simulink model "SVPWMtrialsweird"  (R2015b)
settings: Solver=VariableStepAuto  StartTime=0.0  StopTime=0.05  RelTol=1e-3
libraries: powerlib x29, simulink x1
(part 1 of 2)
settings Model: Creator=hakan  LastModifiedBy=hakan

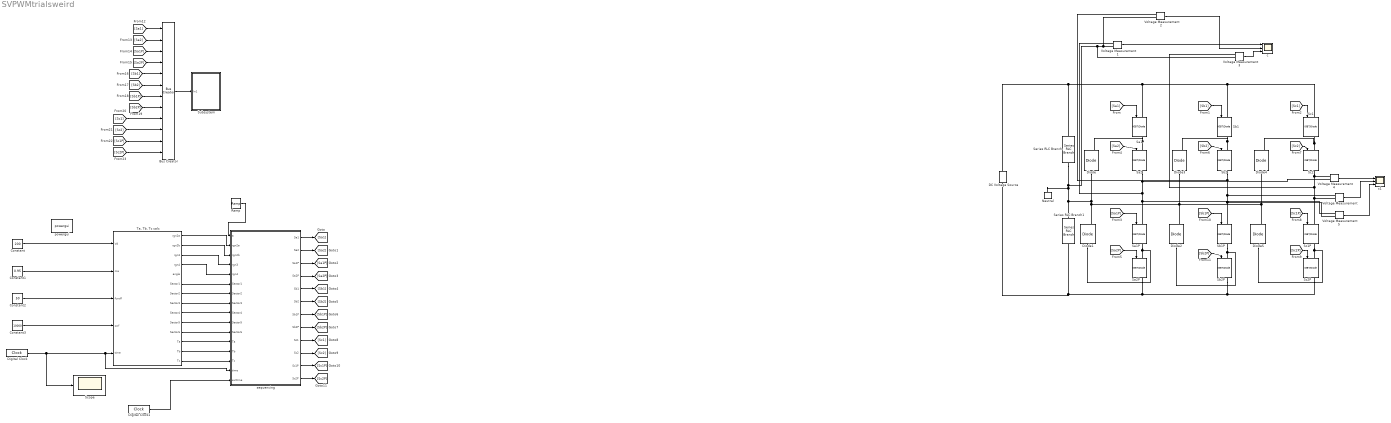
== system SVPWMtrialsweird ==
  Bus Creator : BusCreator  Inputs=12
  Constant : Constant  Value=200
  Constant1 : Constant  Value=0.95
  Constant2 : Constant  Value=50
  Constant3 : Constant  Value=10000  VectorParams1D=off
  DC Voltage Source : powerlib/Electrical Sources/DC Voltage Source  Amplitude=100  Measurements=None
  Digital Clock : DigitalClock  SampleTime=0.00001
  Digital Clock1 : DigitalClock  SampleTime=0.000001
  Diode{,1..5} (6 alike) : powerlib/Power Electronics/Diode  Ron=0.001  Lon=0  Vf=0.8  IC=0  UseSnubber=off  Rs=500  Cs=250e-9  Measurements=on
  Neutral : powerlib/Elements/Neutral  LConnTagsString=a  NodeNumber=10
  Ramp : simulink/Sources/Ramp  slope=1  start=0  X0=0
  "Sa1 " : powerlib/Power Electronics/IGBT//Diode  Ron=1e-3  Rs=1e5  Cs=inf  Measurements=on
  Sa1P : powerlib/Power Electronics/IGBT//Diode  Ron=1e-3  Rs=1e5  Cs=inf  Measurements=on
  Sa2 : powerlib/Power Electronics/IGBT//Diode  Ron=1e-3  Rs=1e5  Cs=inf  Measurements=on
  Sa2P : powerlib/Power Electronics/IGBT//Diode  Ron=1e-3  Rs=1e5  Cs=inf  Measurements=on
  Sb1 : powerlib/Power Electronics/IGBT//Diode  Ron=1e-3  Rs=1e5  Cs=inf  Measurements=on
  Sb1P : powerlib/Power Electronics/IGBT//Diode  Ron=1e-3  Rs=1e5  Cs=inf  Measurements=on
  Sb2 : powerlib/Power Electronics/IGBT//Diode  Ron=1e-3  Rs=1e5  Cs=inf  Measurements=on
  Sb2P : powerlib/Power Electronics/IGBT//Diode  Ron=1e-3  Rs=1e5  Cs=inf  Measurements=on
  Sc1 : powerlib/Power Electronics/IGBT//Diode  Ron=1e-3  Rs=1e5  Cs=inf  Measurements=on
  Sc1P : powerlib/Power Electronics/IGBT//Diode  Ron=1e-3  Rs=1e5  Cs=inf  Measurements=on
  Sc2 : powerlib/Power Electronics/IGBT//Diode  Ron=1e-3  Rs=1e5  Cs=inf  Measurements=on
  Sc2P : powerlib/Power Electronics/IGBT//Diode  Ron=1e-3  Rs=1e5  Cs=inf  Measurements=on
  Scope : Scope
  Series RLC Branch : powerlib/Elements/Series RLC Branch  LConnTagsString=__new0  RConnTagsString=__new0  BranchType=RC  Resistance=1  Inductance=1e-3  SetiL0=off  InitialCurrent=0  Capacitance=1000e-6  Setx0=off  InitialVoltage=0  Measurements=None
  Series RLC Branch1 : powerlib/Elements/Series RLC Branch  LConnTagsString=__new0  RConnTagsString=__new0  BranchType=RC  Resistance=1  Inductance=1e-3  SetiL0=off  InitialCurrent=0  Capacitance=1000e-6  Setx0=off  InitialVoltage=0  Measurements=None
  Subsystem : Subsystem
  "Ta, Tb, Tc calc" : MATLAB Function  TreatAsAtomicUnit=on
  Voltage Measurement{,1..5} (6 alike) : powerlib/Measurements/Voltage Measurement  PhasorSimulation=off  OutputType=Complex  PSBequivalent=0
  c : Scope  NumInputPorts=3
  c1 : Scope  NumInputPorts=3
  powergui : powerlib/powergui  Priority=1  SimulationMode=Continuous  SolverType=Tustin/Backward Euler (TBE)  SampleTime=50e-6  frequency=60  SPID=off  DisableSnubberDevices=off  DisableRonSwitches=off  DisableVfSwitches=off  SwTol=0  DisplayEquations=off  Interpol=off  ExternalGateDelay=off  methode=off  Ts=10  FunctionMessages=off  echomessages=off  HookPort=off  EnableUseOfTLC=off  x0status=blocks  frequencyindice=0  Pbase=100e6  ErrMax=1e-4  Iterations=50  UnitsV=kV  UnitsW=MW  buscounter=0  RestoreLinks=warning  ResistiveCurrentMeasurement=off  Frange=[0:2:500]  Ylog=off  Xlog=on  ShowGrid=off  save=off  variable=ZData  structure=dutycycles  ZoomFFT=off  StartTime=0.0  cycles=1  DisplayStyle=1  fundamental=5000  FreqAxis=off  MaxFrequency=10000  frequencyindicesteady=1  RmsSteady=1  display=off
  sequencing : MATLAB Function  TreatAsAtomicUnit=on
  wires:
  Constant/1 -> "Ta, Tb, Tc calc"/1(Vd)
  Constant1/1 -> "Ta, Tb, Tc calc"/2(ma)
  Constant2/1 -> "Ta, Tb, Tc calc"/3(fundf)
  Constant3/1 -> "Ta, Tb, Tc calc"/4(swf)
  "Ta, Tb, Tc calc"/6(Sector1) -> sequencing/6(Sector1)
  "Ta, Tb, Tc calc"/7(Sector2) -> sequencing/7(Sector2)
  "Ta, Tb, Tc calc"/8(Sector3) -> sequencing/8(Sector3)
  "Ta, Tb, Tc calc"/9(Sector4) -> sequencing/9(Sector4)
  "Ta, Tb, Tc calc"/11(Sector6) -> sequencing/11(Sector6)
  "Ta, Tb, Tc calc"/10(Sector5) -> sequencing/10(Sector5)
  "Ta, Tb, Tc calc"/12(Ta) -> sequencing/12(Ta)
  "Ta, Tb, Tc calc"/13(Tb) -> sequencing/13(Tb)
  "Ta, Tb, Tc calc"/14(Tc) -> sequencing/14(Tc)
  Digital Clock/1 -> sequencing/15(time), "Ta, Tb, Tc calc"/5(time), Scope/1
  Bus Creator/1 -> Subsystem/1(In1)
  sequencing/1(Sa1) -> [Sa1]
  sequencing/2(Sa2) -> [Sa2]
  sequencing/3(Sa1P) -> [Sa1P]
  sequencing/4(Sa2P) -> [Sa2P]
  sequencing/5(Sb1) -> [Sb1]
  sequencing/6(Sb2) -> [Sb2]
  sequencing/7(Sb1P) -> [Sb1P]
  sequencing/8(Sb2P) -> [Sb2P]
  sequencing/9(Sc1) -> [Sc1]
  sequencing/10(Sc2) -> [Sc2]
  sequencing/11(Sc1P) -> [Sc1P]
  sequencing/12(Sc2P) -> [Sc2P]
  [Sa1] -> "Sa1 "/1
  [Sa1P] -> Sa1P/1
  [Sa2] -> Sa2/1
  [Sa2P] -> Sa2P/1
  [Sb1] -> Sb1/1
  [Sb2] -> Sb2/1
  [Sb1P] -> Sb1P/1
  [Sb2P] -> Sb2P/1
  [Sc2P] -> Sc2P/1
  [Sc1P] -> Sc1P/1
  [Sc1] -> Sc1/1
  [Sc2] -> Sc2/1
  [Sa1] -> Bus Creator/1
  [Sa2] -> Bus Creator/2
  [Sa1P] -> Bus Creator/3
  [Sa2P] -> Bus Creator/4
  [Sb1] -> Bus Creator/5
  [Sb2] -> Bus Creator/6
  [Sb1P] -> Bus Creator/7
  [Sb2P] -> Bus Creator/8
  [Sc1] -> Bus Creator/9
  [Sc2] -> Bus Creator/10
  [Sc1P] -> Bus Creator/11
  [Sc2P] -> Bus Creator/12
  Digital Clock1/1 -> sequencing/16(exttime)
  Ramp/1 -> sequencing/1(a)
  "Ta, Tb, Tc calc"/4(rgn4) -> sequencing/5(rgn4)
  "Ta, Tb, Tc calc"/3(rgn3) -> sequencing/4(rgn3)
  "Ta, Tb, Tc calc"/2(rgn2b) -> sequencing/3(rgn2b)
  "Ta, Tb, Tc calc"/1(rgn2a) -> sequencing/2(rgn2a)
  Voltage Measurement3/1 -> c/3
  Voltage Measurement1/1 -> c/1
  Voltage Measurement2/1 -> c/2
  Voltage Measurement4/1 -> c1/1
  Voltage Measurement/1 -> c1/2
  Voltage Measurement5/1 -> c1/3
  connections:
  DC Voltage Source/RConn1 -- Sc1/LConn1 -- Sb1/LConn1 -- "Sa1 "/LConn1 -- Series RLC Branch/LConn1
  DC Voltage Source/LConn1 -- Sb2P/RConn1 -- Sc2P/RConn1 -- Sa2P/RConn1 -- Series RLC Branch1/RConn1
  "Sa1 "/RConn1 -- Diode/RConn1 -- Sa2/LConn1
  Sa2/RConn1 -- Voltage Measurement4/LConn2 -- Voltage Measurement1/LConn1 -- Voltage Measurement5/LConn1 -- Sa1P/LConn1
  Sa1P/RConn1 -- Diode1/LConn1 -- Sa2P/LConn1
  Sb1/RConn1 -- Diode3/RConn1 -- Sb2/LConn1
  Sb2/RConn1 -- Voltage Measurement2/LConn1 -- Voltage Measurement/LConn1 -- Sb1P/LConn1 -- Voltage Measurement5/LConn2
  Sb1P/RConn1 -- Diode2/LConn1 -- Sb2P/LConn1
  Sc1/RConn1 -- Diode4/RConn1 -- Sc2/LConn1
  Sc2/RConn1 -- Voltage Measurement4/LConn1 -- Voltage Measurement3/LConn1 -- Sc1P/LConn1 -- Voltage Measurement/LConn2
  Sc1P/RConn1 -- Diode5/LConn1 -- Sc2P/LConn1
  Diode/LConn1 -- Diode3/LConn1 -- Diode5/RConn1 -- Diode4/LConn1 -- Diode2/RConn1 -- Diode1/RConn1 -- Voltage Measurement2/LConn2 -- Voltage Measurement1/LConn2 -- Voltage Measurement3/LConn2 -- Series RLC Branch/RConn1 -- Neutral/LConn1 -- Series RLC Branch1/LConn1

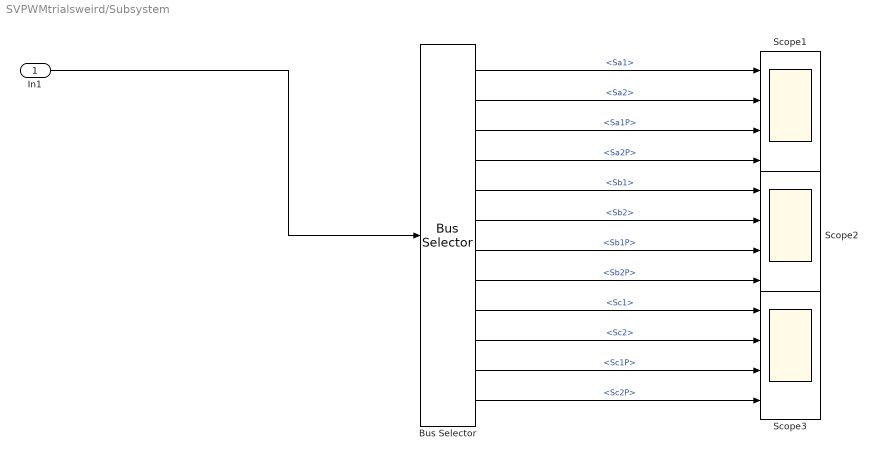
== system SVPWMtrialsweird/Subsystem ==
  In1 : Inport
  Bus Selector : BusSelector  OutputSignals=Sa1,Sa2,Sa1P,Sa2P,Sb1,Sb2,Sb1P,Sb2P,Sc1,Sc2,Sc1P,Sc2P
  Scope1 : Scope  NumInputPorts=4
  Scope2 : Scope  NumInputPorts=4
  Scope3 : Scope  NumInputPorts=4
  wires:
  In1/1 -> Bus Selector/1
  Bus Selector/4 -> Scope1/4  "<Sa2P>"
  Bus Selector/3 -> Scope1/3  "<Sa1P>"
  Bus Selector/2 -> Scope1/2  "<Sa2>"
  Bus Selector/1 -> Scope1/1  "<Sa1>"
  Bus Selector/5 -> Scope2/1  "<Sb1>"
  Bus Selector/6 -> Scope2/2  "<Sb2>"
  Bus Selector/7 -> Scope2/3  "<Sb1P>"
  Bus Selector/8 -> Scope2/4  "<Sb2P>"
  Bus Selector/9 -> Scope3/1  "<Sc1>"
  Bus Selector/12 -> Scope3/4  "<Sc2P>"
  Bus Selector/11 -> Scope3/3  "<Sc1P>"
  Bus Selector/10 -> Scope3/2  "<Sc2>"

== matlab function SVPWMtrialsweird/Ta, Tb, Tc calc ==
  data: rgn2a output; rgn2b output; rgn3 output; rgn4 output; Vd input; ma input; fundf input; angle output; swf input; time input; Sector1 output; Sector2 output; Sector3 output; Sector4 output; Sector5 output; Sector6 output; Ta output; Tb output; Tc output
function [rgn2a, rgn2b, rgn3, rgn4, angle, Sector1, Sector2, Sector3, Sector4, Sector5,Sector6, Ta, Tb, Tc] = fcn(Vd,ma,fundf, swf, time)
% this program works for magnitude of Vref is greater then Vd/3 meaning ma
% must be greater than 1/sqrt(3). for smaller ma's computation is a bit
% more tricky therefore it is omitted for simplicity for now. 
%#ok<*NASGU>
Vref = ma*Vd/sqrt(3); %magnitude of Vref
theta = 2*pi*fundf*time; %angle of Vref
angle = mod(theta, 2*pi);
Ts = 1/swf;
Ta = 0;
Tb = 0;
Tc = 0;
output = 0;
Sector1 = 0; Sector2 = 0; Sector3 = 0; Sector4= 0; Sector5 = 0; Sector6 = 0;
rgn2a = 0 ;rgn2b = 0; rgn3 = 0; rgn4 = 0;
% Sa1=0; Sa2=0; Sa1P=0; Sa2P=0; Sb1=0; Sb2=0; Sb1P=0; Sb2P=0; Sc1=0; Sc2=0; Sc1P=0; Sc2P=0;
anglefrom3to2= 0 ;
%% Sector 1


if (mod(theta, 2*pi)<=pi/3)&&(mod(theta, 2*pi)>0)  % sector 1

    n = 1;
    thetaprime = angle - (n-1)*pi/3;
        for aci = 0:0.00001:pi/3   
            la = sqrt(3)*cos(aci)-sin(aci);
                if (la*ma > 0.99)&&(la*ma<=1)
                    anglefrom3to2 = aci; %leaving angle from region 3 to region 2
                    break
                end
        end

    %anglefrom3to2 = asin(1-1/(sqrt(3)*ma)); 
    anglefrom2to4 = pi/3 - anglefrom3to2; %leaving angle from region 2 to region 4
    if (mod(theta, 2*pi)<=anglefrom3to2) % then sector 1 region 3
        rgn2a = 0 ;rgn2b = 0; rgn3 = 1; rgn4 = 0;
        Ta = Ts*(2-2*ma*sin(pi/3+thetaprime));
        Tb = Ts*2*ma*sin(thetaprime);
        Tc = Ts*(2*ma*sin(pi/3-thetaprime)-1);        
    else if (mod(theta,2*pi)>anglefrom3to2)&&(mod(theta,2*pi)<=anglefrom2to4) % then sector 1 region 2
            if angle<= pi/6 % then 2a
                rgn2a= 1; rgn2b = 0; rgn3 = 0; rgn4=0;
            else % then 2b
                rgn2a= 0; rgn2b = 1; rgn3 = 0; rgn4=0;
            end
            Ta = Ts*(1-2*ma*sin(thetaprime));
            Tb = Ts*(2*ma*sin(pi/3+thetaprime)-1);
            Tc = Ts*(1-2*ma*sin(pi/3-thetaprime));       
        else if (mod(theta,2*pi)>anglefrom2to4) % then sector 1 region 4
               rgn2a = 0 ;rgn2b = 0; rgn3 = 0; rgn4 = 1;
               Ta = Ts*(2*ma*sin(thetaprime)-1);
               Tb = Ts*(2*ma*sin(pi/3-thetaprime));
               Tc = Ts*(2-2*ma*sin(pi/3+thetaprime));               
            end
        end
    end
    Sector1 = 1; Sector2 = 0; Sector3 = 0; Sector4= 0; Sector5 = 0; Sector6 = 0;
end
%% Sector 2


if (mod(theta, 2*pi)<=2*pi/3)&&(mod(theta, 2*pi)>pi/3)  % sector 2
    
    n = 2;
    thetaprime = angle - (n-1)*pi/3;
        for aci = 0:0.00001:pi/3   
            la = sqrt(3)*cos(aci)-sin(aci);
                if (la*ma > 0.99)&&(la*ma<=1)
                    anglefrom3to2 = aci+pi/3; %leaving angle from region 3 to region 2
                    break
                end
        end
    %anglefrom3to2 = pi/3 + asin(1-1/(sqrt(3)*ma));
    anglefrom2to4 = pi/3 + pi/3 - anglefrom3to2;
    if (mod(theta, 2*pi)<=anglefrom3to2) % then sector 2 region 3
        rgn2a = 0 ;rgn2b = 0; rgn3 = 1; rgn4 = 0;
        Ta = Ts*(2-2*ma*sin(pi/3+thetaprime));
        Tb = Ts*2*ma*sin(thetaprime);
        Tc = Ts*(2*ma*sin(pi/3-thetaprime)-1); 
    else if (mod(theta,2*pi)>anglefrom3to2)&&(mod(theta,2*pi)<=anglefrom2to4) % then sector 2 region 2
            if angle<=pi/2 %then 2a
                rgn2a= 1; rgn2b = 0; rgn3 = 0; rgn4=0;
            else % then 2b
                rgn2a= 0; rgn2b = 1; rgn3 = 0; rgn4=0;
            end
            Ta = Ts*(1-2*ma*sin(thetaprime));
            Tb = Ts*(2*ma*sin(pi/3+thetaprime)-1);
            Tc = Ts*(1-2*ma*sin(pi/3-thetaprime)); 
        else if (mod(theta,2*pi)>anglefrom2to4) % then sector 2 region 4
               rgn2a = 0 ;rgn2b = 0; rgn3 = 0; rgn4 = 1;
               Ta = Ts*(2*ma*sin(thetaprime)-1);
               Tb = Ts*(2*ma*sin(pi/3-thetaprime));
               Tc = Ts*(2-2*ma*sin(pi/3+thetaprime)); 
            end
        end
    end
    Sector1 = 0; Sector2 = 1; Sector3 = 0; Sector4= 0; Sector5 = 0; Sector6 = 0;
end
%% Sector 3

if (mod(theta, 2*pi)<=pi)&&(mod(theta, 2*pi)>2*pi/3)  % sector 3
    
    n = 3;
    thetaprime = angle - (n-1)*pi/3;
        for aci = 0:0.00001:pi/3   
            la = sqrt(3)*cos(aci)-sin(aci);
                if (la*ma > 0.99)&&(la*ma<=1)
                    anglefrom3to2 = aci+pi/3+pi/3; %leaving angle from region 3 to region 2
                    break
                end
        end    
    %anglefrom3to2 = 2*pi/3 + asin(1-1/(sqrt(3)*ma));
    anglefrom2to4 = 2*pi/3 + pi/3 - anglefrom3to2;
    if (mod(theta, 2*pi)<=anglefrom3to2) % then sector 3 region 3
        rgn2a = 0 ;rgn2b = 0; rgn3 = 1; rgn4 = 0;
        Ta = Ts*(2-2*ma*sin(pi/3+thetaprime));
        Tb = Ts*2*ma*sin(thetaprime);
        Tc = Ts*(2*ma*sin(pi/3-thetaprime)-1); 
    else if (mod(theta,2*pi)>anglefrom3to2)&&(mod(theta,2*pi)<=anglefrom2to4) % then sector 3 region 2
            if angle<=5*pi/6 %then 2a
                rgn2a= 1; rgn2b = 0; rgn3 = 0; rgn4=0;
            else % then 2b
                rgn2a= 0; rgn2b = 1; rgn3 = 0; rgn4=0;
            end
            Ta = Ts*(1-2*ma*sin(thetaprime));
            Tb = Ts*(2*ma*sin(pi/3+thetaprime)-1);
            Tc = Ts*(1-2*ma*sin(pi/3-thetaprime)); 
        else if (mod(theta,2*pi)>anglefrom2to4) % then sector 3 region 4
                rgn2a = 0 ;rgn2b = 0; rgn3 = 0; rgn4 = 1;
               Ta = Ts*(2*ma*sin(thetaprime)-1);
               Tb = Ts*(2*ma*sin(pi/3-thetaprime));
               Tc = Ts*(2-2*ma*sin(pi/3+thetaprime)); 
            end
        end
    end
    Sector1 = 0; Sector2 = 0; Sector3 = 1; Sector4= 0; Sector5 = 0; Sector6 = 0;
end

%% Sector 4


if (mod(theta, 2*pi)<=4*pi/3)&&(mod(theta, 2*pi)>pi)  % sector 4
    

    n = 4;
    thetaprime = angle - (n-1)*pi/3;
        for aci = 0:0.00001:pi/3   
            la = sqrt(3)*cos(aci)-sin(aci);
                if (la*ma > 0.99)&&(la*ma<=1)
                    anglefrom3to2 = aci+pi/3+pi/3+pi/3; %leaving angle from region 3 to region 2
                    break
                end
        end    
    %anglefrom3to2 = pi + asin(1-1/(sqrt(3)*ma));
    anglefrom2to4 = pi + pi/3 - anglefrom3to2;
    if (mod(theta, 2*pi)<=anglefrom3to2) % then sector 4 region 3
        rgn2a = 0 ;rgn2b = 0; rgn3 = 1; rgn4 = 0;
        Ta = Ts*(2-2*ma*sin(pi/3+thetaprime));
        Tb = Ts*2*ma*sin(thetaprime);
        Tc = Ts*(2*ma*sin(pi/3-thetaprime)-1); 
    else if (mod(theta,2*pi)>anglefrom3to2)&&(mod(theta,2*pi)<=anglefrom2to4) % then sector 4 region 2
            if angle<=7*pi/6 %then 2a
                rgn2a= 1; rgn2b = 0; rgn3 = 0; rgn4=0;
            else % then 2b
                rgn2a= 0; rgn2b = 1; rgn3 = 0; rgn4=0;
            end
            Ta = Ts*(1-2*ma*sin(thetaprime));
            Tb = Ts*(2*ma*sin(pi/3+thetaprime)-1);
            Tc = Ts*(1-2*ma*sin(pi/3-thetaprime));
        else if (mod(theta,2*pi)>anglefrom2to4) % then sector 4 region 4
                rgn2a = 0 ;rgn2b = 0; rgn3 = 0; rgn4 = 1;
               Ta = Ts*(2*ma*sin(thetaprime)-1);
               Tb = Ts*(2*ma*sin(pi/3-thetaprime));
               Tc = Ts*(2-2*ma*sin(pi/3+thetaprime)); 
            end
        end
    end
    Sector1 = 0; Sector2 = 0; Sector3 = 0; Sector4= 1; Sector5 = 0; Sector6 = 0;
end
%% Sector 5 

if (mod(theta, 2*pi)<=5*pi/3)&&(mod(theta, 2*pi)>4*pi/3)  % sector 5
    
    n = 5;
    thetaprime = angle - (n-1)*pi/3;
    %anglefrom3to2 = 4*pi/3 + asin(1-1/(sqrt(3)*ma));
        for aci = 0:0.00001:pi/3   
            la = sqrt(3)*cos(aci)-sin(aci);
                if (la*ma > 0.99)&&(la*ma<=1)
                    anglefrom3to2 = aci+pi/3+pi/3+pi/3+pi/3; %leaving angle from region 3 to region 2
                    break
                end
        end    
    anglefrom2to4 = 4*pi/3 + pi/3 - anglefrom3to2;
    if (mod(theta, 2*pi)<=anglefrom3to2) % then sector 5 region 3
        rgn2a = 0 ;rgn2b = 0; rgn3 = 1; rgn4 = 0;
        Ta = Ts*(2-2*ma*sin(pi/3+thetaprime));
        Tb = Ts*2*ma*sin(thetaprime);
        Tc = Ts*(2*ma*sin(pi/3-thetaprime)-1); 
    else if (mod(theta,2*pi)>anglefrom3to2)&&(mod(theta,2*pi)<=anglefrom2to4) % then sector 5 region 2
            if angle<=3*pi/2 %then 2a
                rgn2a= 1; rgn2b = 0; rgn3 = 0; rgn4=0;
            else % then 2b
                rgn2a= 0; rgn2b = 1; rgn3 = 0; rgn4=0;
            end
            Ta = Ts*(1-2*ma*sin(thetaprime));
            Tb = Ts*(2*ma*sin(pi/3+thetaprime)-1);
            Tc = Ts*(1-2*ma*sin(pi/3-thetaprime));
        else if (mod(theta,2*pi)>anglefrom2to4) % then sector 5 region 4
               rgn2a = 0 ;rgn2b = 0; rgn3 = 0; rgn4 = 1;
               Ta = Ts*(2*ma*sin(thetaprime)-1);
               Tb = Ts*(2*ma*sin(pi/3-thetaprime));
               Tc = Ts*(2-2*ma*sin(pi/3+thetaprime)); 
            end
        end
    end
    Sector1 = 0; Sector2 = 0; Sector3 = 0; Sector4= 0; Sector5 = 1; Sector6 = 0;
end

%% Sector 6 

if (mod(theta, 2*pi)<=2*pi)&&(mod(theta, 2*pi)>5*pi/3)  % sector 6
    
    n = 6;
    thetaprime = angle - (n-1)*pi/3;
        for aci = 0:0.00001:pi/3   
            la = sqrt(3)*cos(aci)-sin(aci);
                if (la*ma > 0.99)&&(la*ma<=1)
                    anglefrom3to2 = aci+pi/3+pi/3+pi/3+pi/3+pi/3; %leaving angle from region 3 to region 2
                    break
                end
        end    
    %anglefrom3to2 = 5*pi/3 + asin(1-1/(sqrt(3)*ma));
    anglefrom2to4 = 5*pi/3 + pi/3 - anglefrom3to2;
    if (mod(theta, 2*pi)<=anglefrom3to2) % then sector 6 region 3
        rgn2a = 0 ;rgn2b = 0; rgn3 = 1; rgn4 = 0;
        Ta = Ts*(2-2*ma*sin(pi/3+thetaprime));
        Tb = Ts*2*ma*sin(thetaprime);
        Tc = Ts*(2*ma*sin(pi/3-thetaprime)-1); 
    else if (mod(theta,2*pi)>anglefrom3to2)&&(mod(theta,2*pi)<=anglefrom2to4) % then sector 6 region 2
            if angle<=11*pi/6 %then 2a
                rgn2a= 1; rgn2b = 0; rgn3 = 0; rgn4=0;
            else % then 2b
                rgn2a= 0; rgn2b = 1; rgn3 = 0; rgn4=0;
            end
            Ta = Ts*(1-2*ma*sin(thetaprime));
            Tb = Ts*(2*ma*sin(pi/3+thetaprime)-1);
            Tc = Ts*(1-2*ma*sin(pi/3-thetaprime));
        else if (mod(theta,2*pi)>anglefrom2to4) % then sector 6 region 4
               rgn2a = 0 ;rgn2b = 0; rgn3 = 0; rgn4 = 1;
               Ta = Ts*(2*ma*sin(thetaprime)-1);
               Tb = Ts*(2*ma*sin(pi/3-thetaprime));
               Tc = Ts*(2-2*ma*sin(pi/3+thetaprime)); 
            end
        end
    end
    Sector1 = 0; Sector2 = 0; Sector3 = 0; Sector4= 0; Sector5 = 0; Sector6 = 1;
end
